simulink model "Hexacopter_ControllerWithNavigation_ver2023b"  (R2023b)
settings: Solver=FixedStepAuto  StartTime=0.0  StopTime=inf  FixedStep=SampleTime  RelTol=1e-3  EnableMultiTasking=on
values from neighbouring files (symbols this model uses):
  SampleTime = 1/250    (= 0.004)    [Init_FLIGHT_Hexacopter.m]    (also in Init_FLIGHT_Hexacopter_fromNCMS.m = 0.01)
undefined symbols (not defined in the file or in its folder): dev, Main, pwm_output0
libraries: px4lib x15, slpidlib x10, px4uORBlib x7, simulink x6, uavalgslib x3, px4Sensorslib x1, simulink_extras x1, sharedutil x1, sharedtransform x1
(part 1 of 3)
settings Model: ExtModeTrigDuration=10  Creator=The MathWorks, Inc.  LastModifiedBy=CNU_UASG
settings SolverCC: PositivePriorityOrder=on  MaxZcPerStep=1
settings OptimizationCC: EnhancedBackFolding=on  PassReuseOutputArgsAs=Individual arguments  ZeroExternalMemoryAtStartup=off  ZeroInternalMemoryAtStartup=off  MaxStackSize=64  OptimizeBlockOrder=speed  DifferentSizesBufferReuse=on  OptimizationCustomize=off  EfficientTunableParamExpr=on
settings DebuggingCC: ParameterTunabilityLossMsg=error
settings HardwareCC: ProdBitPerPointer=32  ProdBitPerSizeT=32  ProdBitPerPtrDiffT=32  ProdLargestAtomicInteger=Long  ProdLargestAtomicFloat=Double  ProdWordSize=32  ProdLongLongMode=on  ProdHWDeviceType=ARM Compatible->ARM Cortex
settings ModelReferenceCC: EnableRefExpFcnMdlSchedulingChecks=on
settings SFSimCC: MATLABDynamicMemAlloc=off  SimTargetLang=C++
settings RTWCC: Description=Embedded Coder  SystemTargetFile=ert.tlc  HardwareBoard=PX4 Cube Orange  TLCOptions="-aInlineSetEventsForThisBaseRateFcn=TLC_FALSE -aSuppressMultiTaskScheduler=TLC_FALSE  -aRateBasedStepFcn=0"  TemplateMakefile=ert_default_tmf  Toolchain=GNU Tools for PX4 Autopilots  TargetLang=C++  DLArmComputeVersion=19.05
settings CodeAppCC: ForceParamTrailComments=on  IgnoreCustomStorageClasses=off  MaxIdLength=63  OperatorAnnotations=on  SimulinkDataObjDesc=on  SFDataObjDesc=on  InsertBlockDesc=on
settings ERTTargetCC: ExtModeTransport=3  ExtModeStaticAlloc=on  ExtModeStaticAllocSize=1024  ExtModeMexFile=ext_xcp  ExtModeIntrfLevel=Level2 - Open

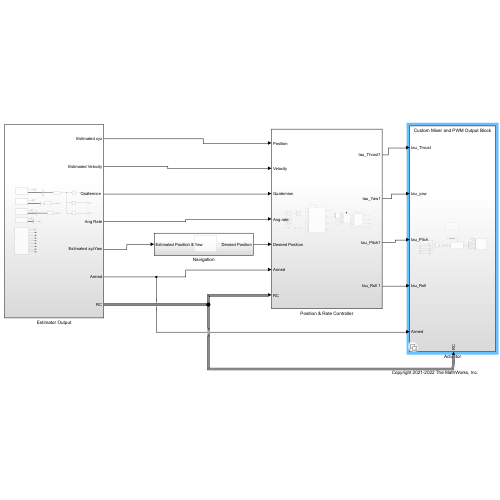
[thumbnail: Simulink's stored preview of the top-level diagram]
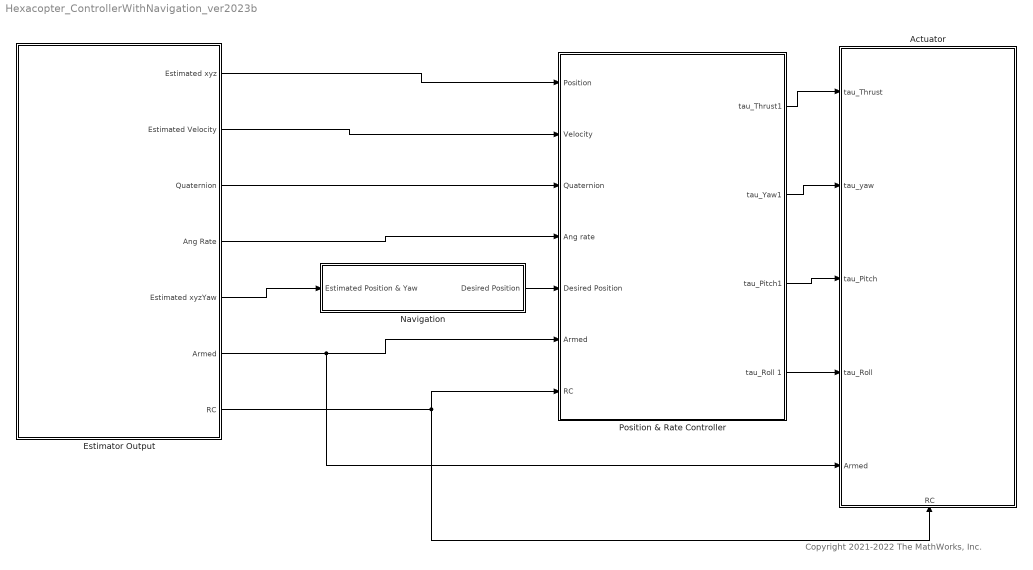
== system Hexacopter_ControllerWithNavigation_ver2023b ==
  note: Copyright 2021-2022 The MathWorks, Inc.
  Actuator : Subsystem  Variant=on
      settings: PortSchema="{\"entries\":[{\"content\":{\"sides\":[{\"content\":{\"connectorIds\":[\"In1\",\"In2\",\"In3\",\"In4\",\"In5\"]},\"type\":\"ConnectorPlacement.EquallySpacedRectSide\",\"uuid\":\"5a9837dd-d0dc-473a-905d-7f1d1e549a1a\"},{\"content\":{\"side\":\"RIGHT\"},\"type\":\"ConnectorPlacement.EquallySpacedRectSide\",\"uuid\":\"ecb902ea-071f-46c7-81c5-182cd0cdfd3c\"},{\"content\":{\"side\":\"TOP\"},\"type\":\"ConnectorPlacement.EquallySpacedRectSide\",\"uuid\":\"3b1ea95c-6dd7-4c60-bfc7-61bcfb955eaa\"},{\"content\":{\"connectorIds\":[\"In6\"],\"side\":\"BOTTOM\"},\"type\":\"ConnectorPlacement.EquallySpacedRectSide\",\"uuid\":\"a3e03740-71d2-4835-8bf3-0b2d7155def1\"}]},\"type\":\"ConnectorPlacement.EquallySpacedConnector\",\"uuid\":\"f571d687-1aa1-4d6b-839e-8b65b8d2b1ab\"}],\"packageUris\":[\"http://schema.mathworks.com/mf0/Connector/R2020b\"],\"version\":\"1.0\"}"
  Estimator Output : Subsystem
  Navigation : Subsystem
  Position & Rate Controller : Subsystem
  wires:
  Estimator Output/5(Estimated xyzYaw) -> Navigation/1(Estimated Position & Yaw)
  Estimator Output/1(Estimated xyz) -> Position & Rate Controller/1(Position)
  Estimator Output/6(Armed) -> Position & Rate Controller/6(Armed), Actuator/5(Armed)
  Estimator Output/2(Estimated Velocity) -> Position & Rate Controller/2(Velocity)
  Estimator Output/7(RC) -> Position & Rate Controller/7(RC), Actuator/6(RC)
  Estimator Output/3("Quaternion ") -> Position & Rate Controller/3(Quaternion)
  Position & Rate Controller/4(tau_Roll 1) -> Actuator/4(tau_Roll)
  Estimator Output/4(Ang Rate) -> Position & Rate Controller/4(Ang rate)
  Navigation/1(Desired Position) -> Position & Rate Controller/5(Desired Position)
  Position & Rate Controller/1(tau_Thrust1) -> Actuator/1(tau_Thrust)
  Position & Rate Controller/2(tau_Yaw1) -> Actuator/2(tau_yaw)
  Position & Rate Controller/3(tau_Pitch1) -> Actuator/3(tau_Pitch)

== system Hexacopter_ControllerWithNavigation_ver2023b/Actuator ==
  tau_Thrust : Inport
  tau_yaw : Inport  Port=2
  tau_Pitch : Inport  Port=3
  tau_Roll : Inport  Port=4
  Armed : Inport  Port=5
  RC : Inport  Port=6
  Custom Mixer and PWM Output Block : Subsystem  VariantControl=useCustomMixer == true
  PX4 Mixer and actuator_controls_0 topic : Subsystem  VariantControl=useCustomMixer == false

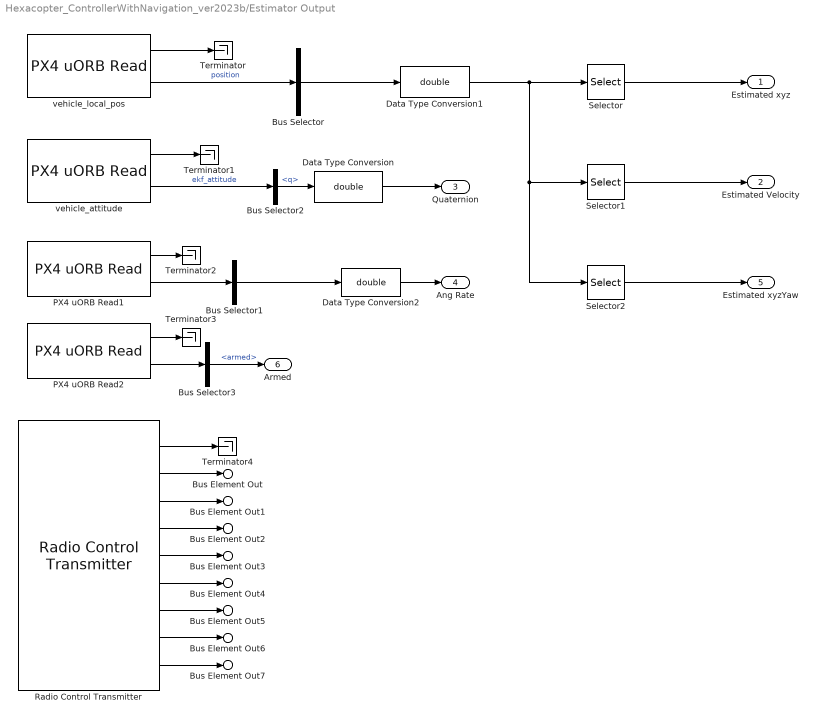
== system Hexacopter_ControllerWithNavigation_ver2023b/Estimator Output ==
  Bus Selector : BusSelector  OutputSignals=x,y,z,vx,vy,vz,heading  OutputAsBus=on
  Bus Selector1 : BusSelector  OutputSignals=rollspeed,pitchspeed,yawspeed  OutputAsBus=on
  Bus Selector2 : BusSelector  OutputSignals=q
  Bus Selector3 : BusSelector  OutputSignals=armed
  Data Type Conversion : DataTypeConversion  OutDataTypeStr=double  SaturateOnIntegerOverflow=off  RndMeth=Floor
  Data Type Conversion1 : DataTypeConversion  OutDataTypeStr=double  SaturateOnIntegerOverflow=off  RndMeth=Floor
  Data Type Conversion2 : DataTypeConversion  OutDataTypeStr=double  SaturateOnIntegerOverflow=off  RndMeth=Floor
  PX4 uORB Read1 : px4uORBlib/PX4 uORB Read  uORBTopic=vehicle_odometry  selectInstance=vehicle_odometry  SampleTime=-1  BlockingMode=off  BlockTimeout=1e-3
  PX4 uORB Read2 : px4uORBlib/PX4 uORB Read  uORBTopic=actuator_armed  selectInstance=actuator_armed  SampleTime=-1  BlockingMode=off  BlockTimeout=1e-3
  Radio Control Transmitter : px4Sensorslib/Radio Control Transmitter  channel1=on  channel2=on  channel3=on  channel4=on  channel5=on  channel6=on  channel7=on  channel8=on  channel_count=off  rssi=off  rc_input_source=off  timestamp_last_signal=off  time_stamp=off  sampleTime=-1  BlockingMode=off  BlockTimeout=5
  Selector : Selector  InputPortWidth=7  IndexOptions=Index vector (dialog)  Indices=[1:3]  OutputSizes=1
  Selector1 : Selector  InputPortWidth=7  IndexOptions=Index vector (dialog)  Indices=[4:6]  OutputSizes=1
  Selector2 : Selector  InputPortWidth=7  IndexOptions=Index vector (dialog)  Indices=[1 2 3 7]  OutputSizes=1
  Terminator{,1..4} (5 alike) : Terminator
  vehicle_attitude : px4uORBlib/PX4 uORB Read  uORBTopic=vehicle_attitude  selectInstance=vehicle_attitude  SampleTime=-1  BlockingMode=off  BlockTimeout=1e-3
  vehicle_local_pos : px4uORBlib/PX4 uORB Read  uORBTopic=vehicle_local_position  selectInstance=vehicle_local_position  SampleTime=-1  BlockingMode=off  BlockTimeout=1e-3
  Estimated xyz : Outport
  Estimated Velocity : Outport  Port=2
  "Quaternion " : Outport  Port=3
  Ang Rate : Outport  Port=4
  Estimated xyzYaw : Outport  Port=5
  Armed : Outport  Port=6
  Bus Element Out : Outport  Port=7  PortName=RC  Element=roll
  Bus Element Out1 : Outport  Port=7  PortName=RC  Element=pitch
  Bus Element Out2 : Outport  Port=7  PortName=RC  Element=throttle
  Bus Element Out3 : Outport  Port=7  PortName=RC  Element=yaw
  Bus Element Out4 : Outport  Port=7  PortName=RC  Element=arm
  Bus Element Out5 : Outport  Port=7  PortName=RC  Element=mode
  Bus Element Out6 : Outport  Port=7  PortName=RC  Element=kill
  Bus Element Out7 : Outport  Port=7  PortName=RC  Element=injectFault
  wires:
  Data Type Conversion/1 -> "Quaternion "/1
  Bus Selector2/1 -> Data Type Conversion/1  "<q>"
  vehicle_local_pos/2 -> Bus Selector/1  "position"
  Data Type Conversion1/1 -> Selector1/1, Selector2/1, Selector/1
  Selector2/1 -> Estimated xyzYaw/1
  vehicle_attitude/1 -> Terminator1/1
  vehicle_attitude/2 -> Bus Selector2/1  "ekf_attitude"
  vehicle_local_pos/1 -> Terminator/1
  Selector/1 -> Estimated xyz/1
  Selector1/1 -> Estimated Velocity/1
  Bus Selector/1 -> Data Type Conversion1/1
  PX4 uORB Read1/1 -> Terminator2/1
  Data Type Conversion2/1 -> Ang Rate/1
  PX4 uORB Read1/2 -> Bus Selector1/1
  PX4 uORB Read2/1 -> Terminator3/1
  Bus Selector3/1 -> Armed/1  "<armed>"
  PX4 uORB Read2/2 -> Bus Selector3/1
  Bus Selector1/1 -> Data Type Conversion2/1
  Radio Control Transmitter/1 -> Terminator4/1
  Radio Control Transmitter/2 -> Bus Element Out/1
  Radio Control Transmitter/3 -> Bus Element Out1/1
  Radio Control Transmitter/4 -> Bus Element Out2/1
  Radio Control Transmitter/5 -> Bus Element Out3/1
  Radio Control Transmitter/6 -> Bus Element Out4/1
  Radio Control Transmitter/7 -> Bus Element Out5/1
  Radio Control Transmitter/8 -> Bus Element Out6/1
  Radio Control Transmitter/9 -> Bus Element Out7/1

== system Hexacopter_ControllerWithNavigation_ver2023b/Navigation ==
  Estimated Position & Yaw : Inport
  Quadcopter Navigation Algorithm : Subsystem  Variant=on
  Desired Position : Outport
  wires:
  Quadcopter Navigation Algorithm/1(Desired Position) -> Desired Position/1
  Estimated Position & Yaw/1 -> Quadcopter Navigation Algorithm/1(Current Position)

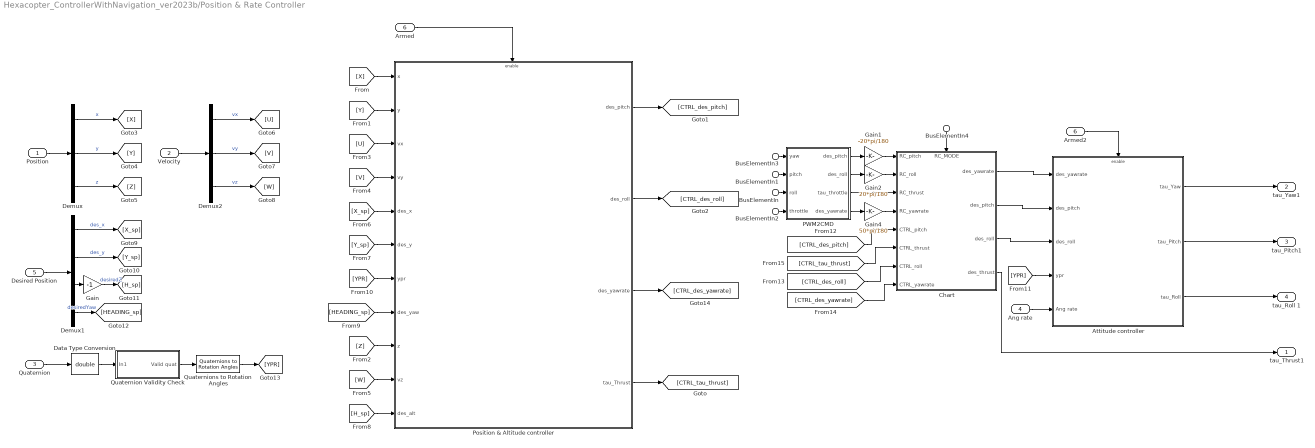
== system Hexacopter_ControllerWithNavigation_ver2023b/Position & Rate Controller ==
  Position : Inport
  Velocity : Inport  Port=2
  Quaternion : Inport  Port=3
  Ang rate : Inport  Port=4
  Desired Position : Inport  Port=5
  Armed : Inport  Port=6
  BusElementIn : Inport  Port=7  PortName=RC  Element=roll
  BusElementIn1 : Inport  Port=7  PortName=RC  Element=pitch
  BusElementIn2 : Inport  Port=7  PortName=RC  Element=throttle
  BusElementIn3 : Inport  Port=7  PortName=RC  Element=yaw
  BusElementIn4 : Inport  Port=7  PortName=RC  Element=mode
  Armed2 : InportShadow  Port=6
  Attitude controller : Subsystem
  Chart : Stateflow chart  TreatAsAtomicUnit=on
      settings: PortSchema="{\"entries\":[{\"content\":{\"sides\":[{\"content\":{\"connectorIds\":[\"In1\",\"In2\",\"In3\",\"In4\",\"In5\",\"In6\",\"In7\",\"In8\"]},\"type\":\"ConnectorPlacement.EquallySpacedRectSide\",\"uuid\":\"1fe492af-6951-4977-8845-2827c5fffa90\"},{\"content\":{\"connectorIds\":[\"Out4\",\"Out1\",\"Out2\",\"Out3\"],\"side\":\"RIGHT\"},\"type\":\"ConnectorPlacement.EquallySpacedRectSide\",\"uuid\":\"b9696a80-46ec-4207-8603-554fdadc7482\"},{\"content\":{\"connectorIds\":[\"In9\"],\"side\":\"TOP\"},\"type\":\"ConnectorPlacement.EquallySpacedRectSide\",\"uuid\":\"36570070-de44-4c7d-99d4-966866a3d58a\"}]},\"type\":\"ConnectorPlacement.EquallySpacedConnector\",\"uuid\":\"856ffff0-a9f0-4cf1-b884-50c3ab6b91f5\"}],\"packageUris\":[\"http://schema.mathworks.com/mf0/Connector/R2020b\"],\"version\":\"1.0\"}"
  Data Type Conversion : DataTypeConversion  OutDataTypeStr=double  SaturateOnIntegerOverflow=off  RndMeth=Floor
  Demux : Demux  Outputs=3
  Demux1 : Demux
  Demux2 : Demux  Outputs=3
  Gain : Gain  Gain=-1
  Gain1 : Gain  Gain=-20*pi/180
  Gain2 : Gain  Gain=20*pi/180
  Gain4 : Gain  Gain=50*pi/180
  PWM2CMD : Subsystem
  Position & Altitude controller : Subsystem
  Quaternion Validity Check : Subsystem
  Quaternions to Rotation Angles : sharedtransform/Quaternions to Rotation Angles  rotationOrder=ZYX  aMode=aMode
  tau_Thrust1 : Outport
  tau_Yaw1 : Outport  Port=2
  tau_Pitch1 : Outport  Port=3
  tau_Roll 1 : Outport  Port=4
  wires:
  Attitude controller/1(tau_Yaw) -> tau_Yaw1/1
  Position & Altitude controller/1(des_pitch) -> [CTRL_des_pitch]
  Data Type Conversion/1 -> Quaternion Validity Check/1(In1)
  Quaternion Validity Check/1(Valid quat) -> Quaternions to Rotation Angles/1
  Position/1 -> Demux/1
  Desired Position/1 -> Demux1/1
  Velocity/1 -> Demux2/1
  Quaternion/1 -> Data Type Conversion/1
  Attitude controller/2(tau_Pitch) -> tau_Pitch1/1
  Attitude controller/3(tau_Roll) -> tau_Roll 1/1
  Demux1/3 -> Gain/1
  Position & Altitude controller/2(des_roll) -> [CTRL_des_roll]
  Ang rate/1 -> Attitude controller/5(Ang rate)
  Demux/1 -> [X]  "x"
  Demux/2 -> [Y]  "y"
  Demux/3 -> [Z]  "z"
  [Y] -> Position & Altitude controller/2(y)
  [X] -> Position & Altitude controller/1(x)
  Demux2/1 -> [U]  "vx"
  Demux2/2 -> [V]  "vy"
  Demux2/3 -> [W]  "vz"
  [U] -> Position & Altitude controller/3(vx)
  [V] -> Position & Altitude controller/4(vy)
  Demux1/1 -> [X_sp]  "des_x"
  Demux1/2 -> [Y_sp]  "des_y"
  Gain/1 -> [H_sp]  "desiredZ"
  [Y_sp] -> Position & Altitude controller/6(des_y)
  [X_sp] -> Position & Altitude controller/5(des_x)
  Demux1/4 -> [HEADING_sp]  "desiredYaw"
  [HEADING_sp] -> Position & Altitude controller/8(des_yaw)
  Quaternions to Rotation Angles/1 -> [YPR]
  [YPR] -> Position & Altitude controller/7(ypr)
  [YPR] -> Attitude controller/4(ypr)
  Position & Altitude controller/3(des_yawrate) -> [CTRL_des_yawrate]
  Chart/4(des_yawrate) -> Attitude controller/1(des_yawrate)
  Chart/1(des_pitch) -> Attitude controller/2(des_pitch)
  Chart/2(des_roll) -> Attitude controller/3(des_roll)
  Chart/3(des_thrust) -> tau_Thrust1/1
  [Z] -> Position & Altitude controller/9(z)
  [W] -> Position & Altitude controller/10(vz)
  [H_sp] -> Position & Altitude controller/11(des_alt)
  Position & Altitude controller/4(tau_Thrust) -> [CTRL_tau_thrust]
  [CTRL_des_pitch] -> Chart/5(CTRL_pitch)
  [CTRL_des_roll] -> Chart/7(CTRL_roll)
  [CTRL_des_yawrate] -> Chart/8(CTRL_yawrate)
  [CTRL_tau_thrust] -> Chart/6(CTRL_thrust)
  BusElementIn3/1 -> PWM2CMD/1(yaw)
  BusElementIn1/1 -> PWM2CMD/2(pitch)
  BusElementIn/1 -> PWM2CMD/3(roll)
  BusElementIn2/1 -> PWM2CMD/4(throttle)
  BusElementIn4/1 -> Chart/9(RC_MODE)
  PWM2CMD/1(des_pitch) -> Gain1/1
  PWM2CMD/4(des_yawrate) -> Gain4/1
  Gain1/1 -> Chart/1(RC_pitch)
  PWM2CMD/3(tau_throttle) -> Chart/3(RC_thrust)
  Gain4/1 -> Chart/4(RC_yawrate)
  PWM2CMD/2(des_roll) -> Gain2/1
  Gain2/1 -> Chart/2(RC_roll)
  Armed/1 -> Position & Altitude controller/Enable
  Armed2/1 -> Attitude controller/Enable

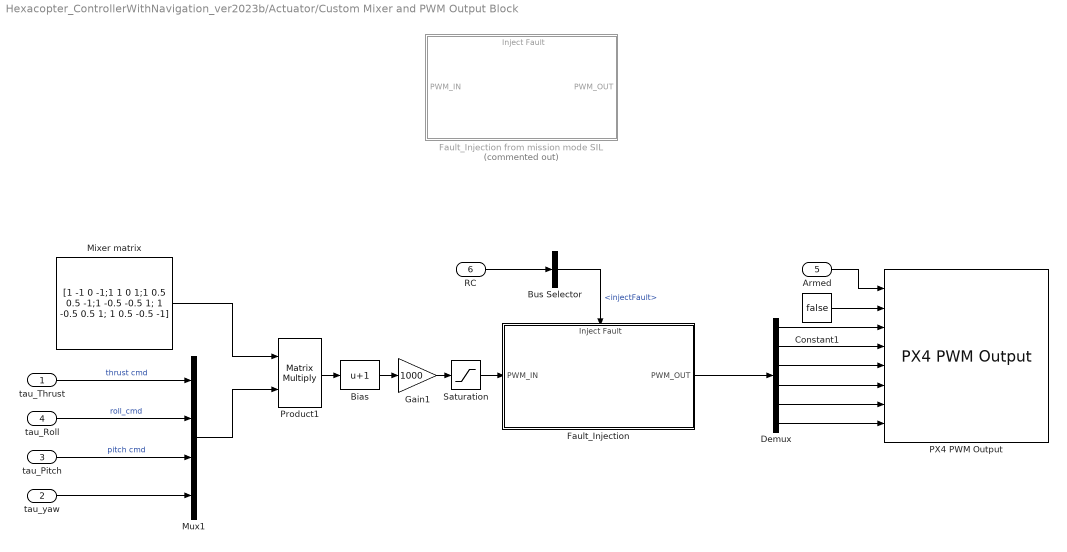
== system Hexacopter_ControllerWithNavigation_ver2023b/Actuator/Custom Mixer and PWM Output Block ==
  tau_Thrust : Inport
  tau_yaw : Inport  Port=2
  tau_Pitch : Inport  Port=3
  tau_Roll : Inport  Port=4
  Armed : Inport  Port=5
  RC : Inport  Port=6
  Bias : Bias  Bias=1  SaturateOnIntegerOverflow=off
  Bus Selector : BusSelector  OutputSignals=injectFault
  Constant1 : Constant  Value=false
  Demux : Demux  Outputs=6
  Fault_Injection : Subsystem  VariantControl=(default)
      settings: PortSchema="{\"entries\":[{\"content\":{\"sides\":[{\"content\":{\"connectorIds\":[\"In1\"]},\"type\":\"ConnectorPlacement.EquallySpacedRectSide\",\"uuid\":\"fab26c65-8d77-46b7-b375-2033d08e8306\"},{\"content\":{\"connectorIds\":[\"Out1\"],\"side\":\"RIGHT\"},\"type\":\"ConnectorPlacement.EquallySpacedRectSide\",\"uuid\":\"bc3f50bd-e170-4b75-8089-4f92da68e83e\"},{\"content\":{\"connectorIds\":[\"In2\"],\"side\":\"TOP\"},\"type\":\"ConnectorPlacement.EquallySpacedRectSide\",\"uuid\":\"873ada90-6f93-48ab-a701-a52d28357753\"}]},\"type\":\"ConnectorPlacement.EquallySpacedConnector\",\"uuid\":\"201be8b3-bff4-4924-8e0c-28e5fee33d1c\"}],\"packageUris\":[\"http://schema.mathworks.com/mf0/Connector/R2020b\"],\"version\":\"1.0\"}"
  Fault_Injection from mission mode SIL : Subsystem  Commented=on
      settings: PortSchema="{\"entries\":[{\"content\":{\"sides\":[{\"content\":{\"connectorIds\":[\"In1\"]},\"type\":\"ConnectorPlacement.EquallySpacedRectSide\",\"uuid\":\"fab26c65-8d77-46b7-b375-2033d08e8306\"},{\"content\":{\"connectorIds\":[\"Out1\"],\"side\":\"RIGHT\"},\"type\":\"ConnectorPlacement.EquallySpacedRectSide\",\"uuid\":\"bc3f50bd-e170-4b75-8089-4f92da68e83e\"},{\"content\":{\"connectorIds\":[\"In2\"],\"side\":\"TOP\"},\"type\":\"ConnectorPlacement.EquallySpacedRectSide\",\"uuid\":\"873ada90-6f93-48ab-a701-a52d28357753\"}]},\"type\":\"ConnectorPlacement.EquallySpacedConnector\",\"uuid\":\"201be8b3-bff4-4924-8e0c-28e5fee33d1c\"}],\"packageUris\":[\"http://schema.mathworks.com/mf0/Connector/R2020b\"],\"version\":\"1.0\"}"
  Gain1 : Gain  Gain=1000  OutDataTypeStr=uint16
  Mixer matrix : Constant  Value=[1 -1 0 -1;1 1 0 1;1 0.5 0.5 -1;1 -0.5 -0.5 1; 1 -0.5 0.5 1; 1 0.5 -0.5 -1]  OutDataTypeStr=Inherit: Inherit via back propagation  SampleTime=-1
  Mux1 : Mux
  PX4 PWM Output : px4lib/PX4 PWM Output  pwmDevice=Main (/dev/pwm_output0)  pwmChannel1_=on  pwmChannel2_=on  pwmChannel3_=on  pwmChannel4_=on  pwmChannel5_=on  pwmChannel6_=on  pwmChannel7_=off  pwmChannel8_=off  forceTerminateFailsafe=off  outputErrorStatus=off
  Product1 : Product  Multiplication=Matrix(*)  RndMeth=Zero
  Saturation : Saturate  UpperLimit=2000  LowerLimit=1000
  wires:
  Demux/1 -> PX4 PWM Output/3
  Demux/2 -> PX4 PWM Output/4
  Gain1/1 -> Saturation/1
  Mux1/1 -> Product1/2
  Mixer matrix/1 -> Product1/1
  tau_Thrust/1 -> Mux1/1  "thrust cmd"
  Constant1/1 -> PX4 PWM Output/2
  Demux/3 -> PX4 PWM Output/5
  Armed/1 -> PX4 PWM Output/1
  Product1/1 -> Bias/1
  Demux/4 -> PX4 PWM Output/6
  Bias/1 -> Gain1/1
  tau_Roll/1 -> Mux1/2  "roll_cmd"
  tau_Pitch/1 -> Mux1/3  "pitch cmd"
  tau_yaw/1 -> Mux1/4
  Demux/5 -> PX4 PWM Output/7
  Demux/6 -> PX4 PWM Output/8
  RC/1 -> Bus Selector/1
  Saturation/1 -> Fault_Injection/1(PWM_IN)
  Fault_Injection/1(PWM_OUT) -> Demux/1
  Bus Selector/1 -> Fault_Injection/2(Inject Fault)  "<injectFault>"

== system Hexacopter_ControllerWithNavigation_ver2023b/Actuator/PX4 Mixer and actuator_controls_0 topic ==
  tau_Thrust : Inport
  tau_yaw : Inport  Port=2
  tau_Pitch : Inport  Port=3
  tau_Roll : Inport  Port=4
  Armed : Inport  Port=5
  RC : Inport  Port=6
  Bus Assignment : BusAssignment  AssignedSignals=control
  Constant : Constant  Value=zeros(4,1)
  Data Type Conversion : DataTypeConversion  SaturateOnIntegerOverflow=off  RndMeth=Floor
  Mux : Mux  Inputs=5
  PX4 uORB Message : px4uORBlib/PX4 uORB Message  uORBTopic=actuator_controls  SampleTime=inf  selectInstance=vehicle_gps_position
  PX4 uORB Write : px4uORBlib/PX4 uORB Write  uORBTopic=actuator_controls  selectInstance=actuator_controls_0  MessageQueueLen=1
  Terminator : Terminator
  wires:
  Bus Assignment/1 -> PX4 uORB Write/1
  tau_yaw/1 -> Mux/3
  Data Type Conversion/1 -> Bus Assignment/2
  tau_Roll/1 -> Mux/1  "roll_cmd"
  PX4 uORB Message/1 -> Bus Assignment/1
  Mux/1 -> Data Type Conversion/1
  Constant/1 -> Mux/5
  tau_Pitch/1 -> Mux/2  "pitch cmd"
  tau_Thrust/1 -> Mux/4  "thrust cmd"
  Armed/1 -> Terminator/1

== system Hexacopter_ControllerWithNavigation_ver2023b/Navigation/Quadcopter Navigation Algorithm ==
  Current Position : Inport
  Manual Waypoints : Subsystem  VariantControl=guidanceType == 3
  Manual Waypoints from Simulink Dashboard : Subsystem  VariantControl=guidanceType == 2
  Path Correction from Onboard Computer : Subsystem  VariantControl=guidanceType == 1
  Read waypoint from QGroundControl Mission : Subsystem  VariantControl=guidanceType == 0
  Desired Position : Outport

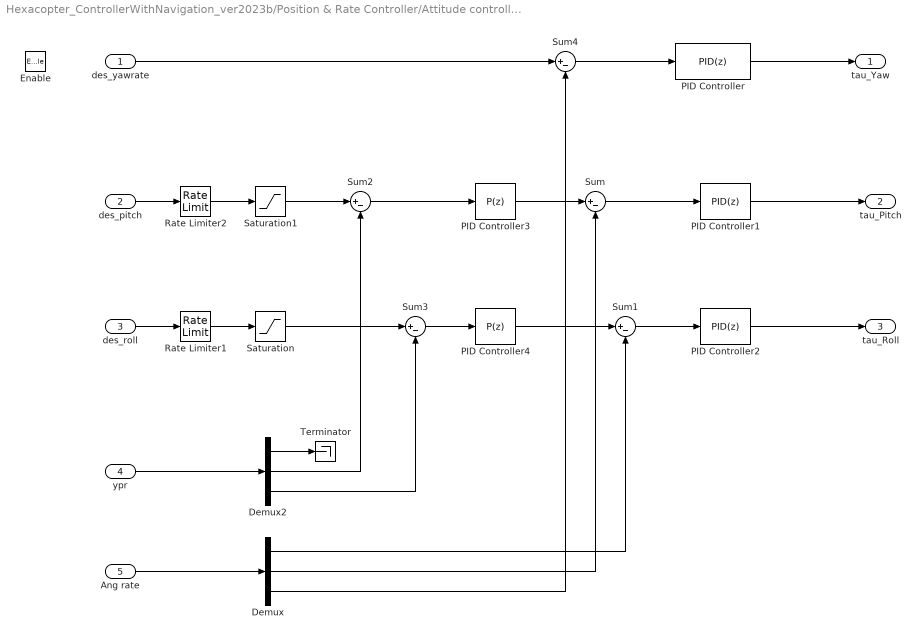
== system Hexacopter_ControllerWithNavigation_ver2023b/Position & Rate Controller/Attitude controller ==
  des_yawrate : Inport
  des_pitch : Inport  Port=2
  des_roll : Inport  Port=3
  ypr : Inport  Port=4
  Ang rate : Inport  Port=5
  Enable : EnablePort
  Demux : Demux  Outputs=3
  Demux2 : Demux  Outputs=3
  PID Controller : slpidlib/PID Controller  Controller=PID  Form=Parallel  TimeDomain=Discrete-time  UseExternalTs=off  SampleTime=-1  IntegratorMethod=Forward Euler  FilterMethod=Forward Euler  ControllerParametersSource=internal  P=0.2/10  I=0.1/10  UseKiTs=on  D=0  N=100  UseFilter=on  TunerSelectOption=Transfer Function Based (PID Tuner App)  InitialConditionSource=internal  InitialConditionForIntegrator=0  InitialConditionForFilter=0  DifferentiatorICPrevScaledInput=0  ExternalReset=none  TrackingMode=off  Kt=1  LimitOutput=on  SatLimitsSource=internal  UpperSaturationLimit=0.1  LowerSaturationLimit=-0.1  LinearizeAsGain=on  AntiWindupMode=clamping  Kb=1  LimitIntegrator=off  UpperIntegratorSaturationLimit=inf  LowerIntegratorSaturationLimit=-inf  POutMin=[]  POutMax=[]  IOutMin=[]  IOutMax=[]  DOutMin=[]  DOutMax=[]  NOutMin=[]  NOutMax=[]  SumOutMin=[]  SumOutMax=[]  SaturationOutMin=[]  SaturationOutMax=[]  PParamMin=[]  PParamMax=[]  IParamMin=[]  IParamMax=[]  DParamMin=[]  DParamMax=[]  NParamMin=[]  NParamMax=[]  KbParamMin=[]  KbParamMax=[]  KtParamMin=[]  KtParamMax=[]  KbOutMin=[]  KbOutMax=[]  KtOutMin=[]  KtOutMax=[]  IntegratorOutMin=[]  IntegratorOutMax=[]  FilterOutMin=[]  FilterOutMax=[]  SumI1OutMin=[]  SumI1OutMax=[]  SumI2OutMin=[]  SumI2OutMax=[]  SumI3OutMin=[]  SumI3OutMax=[]  SumI4OutMin=[]  SumI4OutMax=[]  SumDOutMin=[]  SumDOutMax=[]  DifferentiatorOutMin=[]  DifferentiatorOutMax=[]  FilterDiffOutCoefMin=[]  FilterDiffOutCoefMax=[]  ReciprocalOutMin=[]  ReciprocalOutMax=[]  SumDenOutMin=[]  SumDenOutMax=[]  SumNumOutMin=[]  SumNumOutMax=[]  DivideOutMin=[]  DivideOutMax=[]  UdiffTsProdOutMin=[]  UdiffTsProdOutMax=[]  NTsProdOutMin=[]  NTsProdOutMax=[]  UintegralTsProdOutMin=[]  UintegralTsProdOutMax=[]  UngainTsProdOutMin=[]  UngainTsProdOutMax=[]  ClampingZeroOutDataTypeStr=Inherit: Inherit via back propagation  ClampingZeroOutMin=[]  ClampingZeroOutMax=[]  FilterDenConstantOutDataTypeStr=Inherit: Inherit via back propagation  FilterDenConstantOutMin=[]  FilterDenConstantOutMax=[]  PCopyOutDataTypeStr=Inherit: Inherit via back propagation  PCopyOutMin=[]  PCopyOutMax=[]  NCopyOutDataTypeStr=Inherit: Inherit via back propagation  NCopyOutMin=[]  NCopyOutMax=[]  IntegratorContinuousStateAttributes=''  IntegratorStateMustResolveToSignalObject=off  IntegratorRTWStateStorageClass=Auto  FilterContinuousStateAttributes=''  FilterStateMustResolveToSignalObject=off  FilterRTWStateStorageClass=Auto  ParallelPVariant=InternalParameters  IdealPVariant=Disabled  IVariant=InternalParameters  DVariant=InternalParameters  IntegratorVariant=Discrete  SatVariant=Enabled  AWVariant=DiscClampingParallel  PCopyVariant=Disabled  TRVariant=Disabled  FdbkBlocksVariant=Forward  IdealPFdbkVariant=Disabled  SatFdbkVariant=Disabled  DerivativeFilterVariant=ForwardEulerFilter  NVariant=InternalParameters  NCopyVariant=Disabled  FilterICVariant=InternalICsFilter  IntegratorICVariant=InternalICs  ExternalResetVariant=Disabled  TRSumVariant=Passthrough  SumFdbkVariant=Disabled  SumVariant=Sum_PID  TsampFilterVariant=InternalTs  TsampNgainVariant=Passthrough  TsampIntegralVariant=Disabled_SignalSpec  ExternalSaturationOutDataTypeStr=Inherit: Same as second input
  PID Controller1 : slpidlib/PID Controller  Controller=PID  Form=Parallel  TimeDomain=Discrete-time  UseExternalTs=off  SampleTime=-1  IntegratorMethod=Forward Euler  FilterMethod=Forward Euler  ControllerParametersSource=internal  P=0.15/5  I=0.2/5  UseKiTs=on  D=0.003/5  N=50  UseFilter=on  TunerSelectOption=Transfer Function Based (PID Tuner App)  InitialConditionSource=internal  InitialConditionForIntegrator=0  InitialConditionForFilter=0  DifferentiatorICPrevScaledInput=0  ExternalReset=none  TrackingMode=off  Kt=1  LimitOutput=on  SatLimitsSource=internal  UpperSaturationLimit=0.2  LowerSaturationLimit=-0.2  LinearizeAsGain=on  AntiWindupMode=clamping  Kb=1  LimitIntegrator=off  UpperIntegratorSaturationLimit=inf  LowerIntegratorSaturationLimit=-inf  POutMin=[]  POutMax=[]  IOutMin=[]  IOutMax=[]  DOutMin=[]  DOutMax=[]  NOutMin=[]  NOutMax=[]  SumOutMin=[]  SumOutMax=[]  SaturationOutMin=[]  SaturationOutMax=[]  PParamMin=[]  PParamMax=[]  IParamMin=[]  IParamMax=[]  DParamMin=[]  DParamMax=[]  NParamMin=[]  NParamMax=[]  KbParamMin=[]  KbParamMax=[]  KtParamMin=[]  KtParamMax=[]  KbOutMin=[]  KbOutMax=[]  KtOutMin=[]  KtOutMax=[]  IntegratorOutMin=[]  IntegratorOutMax=[]  FilterOutMin=[]  FilterOutMax=[]  SumI1OutMin=[]  SumI1OutMax=[]  SumI2OutMin=[]  SumI2OutMax=[]  SumI3OutMin=[]  SumI3OutMax=[]  SumI4OutMin=[]  SumI4OutMax=[]  SumDOutMin=[]  SumDOutMax=[]  DifferentiatorOutMin=[]  DifferentiatorOutMax=[]  FilterDiffOutCoefMin=[]  FilterDiffOutCoefMax=[]  ReciprocalOutMin=[]  ReciprocalOutMax=[]  SumDenOutMin=[]  SumDenOutMax=[]  SumNumOutMin=[]  SumNumOutMax=[]  DivideOutMin=[]  DivideOutMax=[]  UdiffTsProdOutMin=[]  UdiffTsProdOutMax=[]  NTsProdOutMin=[]  NTsProdOutMax=[]  UintegralTsProdOutMin=[]  UintegralTsProdOutMax=[]  UngainTsProdOutMin=[]  UngainTsProdOutMax=[]  ClampingZeroOutDataTypeStr=Inherit: Inherit via back propagation  ClampingZeroOutMin=[]  ClampingZeroOutMax=[]  FilterDenConstantOutDataTypeStr=Inherit: Inherit via back propagation  FilterDenConstantOutMin=[]  FilterDenConstantOutMax=[]  PCopyOutDataTypeStr=Inherit: Inherit via back propagation  PCopyOutMin=[]  PCopyOutMax=[]  NCopyOutDataTypeStr=Inherit: Inherit via back propagation  NCopyOutMin=[]  NCopyOutMax=[]  IntegratorContinuousStateAttributes=''  IntegratorStateMustResolveToSignalObject=off  IntegratorRTWStateStorageClass=Auto  FilterContinuousStateAttributes=''  FilterStateMustResolveToSignalObject=off  FilterRTWStateStorageClass=Auto  ParallelPVariant=InternalParameters  IdealPVariant=Disabled  IVariant=InternalParameters  DVariant=InternalParameters  IntegratorVariant=Discrete  SatVariant=Enabled  AWVariant=DiscClampingParallel  PCopyVariant=Disabled  TRVariant=Disabled  FdbkBlocksVariant=Forward  IdealPFdbkVariant=Disabled  SatFdbkVariant=Disabled  DerivativeFilterVariant=ForwardEulerFilter  NVariant=InternalParameters  NCopyVariant=Disabled  FilterICVariant=InternalICsFilter  IntegratorICVariant=InternalICs  ExternalResetVariant=Disabled  TRSumVariant=Passthrough  SumFdbkVariant=Disabled  SumVariant=Sum_PID  TsampFilterVariant=InternalTs  TsampNgainVariant=Passthrough  TsampIntegralVariant=Disabled_SignalSpec  ExternalSaturationOutDataTypeStr=Inherit: Same as second input
  PID Controller2 : slpidlib/PID Controller  Controller=PID  Form=Parallel  TimeDomain=Discrete-time  UseExternalTs=off  SampleTime=-1  IntegratorMethod=Forward Euler  FilterMethod=Forward Euler  ControllerParametersSource=internal  P=0.15/5  I=0.2/5  UseKiTs=off  D=0.003/5  N=50  UseFilter=on  TunerSelectOption=Transfer Function Based (PID Tuner App)  InitialConditionSource=internal  InitialConditionForIntegrator=0  InitialConditionForFilter=0  DifferentiatorICPrevScaledInput=0  ExternalReset=none  TrackingMode=off  Kt=1  LimitOutput=on  SatLimitsSource=internal  UpperSaturationLimit=0.2  LowerSaturationLimit=-0.2  LinearizeAsGain=on  AntiWindupMode=clamping  Kb=1  LimitIntegrator=off  UpperIntegratorSaturationLimit=inf  LowerIntegratorSaturationLimit=-inf  POutMin=[]  POutMax=[]  IOutMin=[]  IOutMax=[]  DOutMin=[]  DOutMax=[]  NOutMin=[]  NOutMax=[]  SumOutMin=[]  SumOutMax=[]  SaturationOutMin=[]  SaturationOutMax=[]  PParamMin=[]  PParamMax=[]  IParamMin=[]  IParamMax=[]  DParamMin=[]  DParamMax=[]  NParamMin=[]  NParamMax=[]  KbParamMin=[]  KbParamMax=[]  KtParamMin=[]  KtParamMax=[]  KbOutMin=[]  KbOutMax=[]  KtOutMin=[]  KtOutMax=[]  IntegratorOutMin=[]  IntegratorOutMax=[]  FilterOutMin=[]  FilterOutMax=[]  SumI1OutMin=[]  SumI1OutMax=[]  SumI2OutMin=[]  SumI2OutMax=[]  SumI3OutMin=[]  SumI3OutMax=[]  SumI4OutMin=[]  SumI4OutMax=[]  SumDOutMin=[]  SumDOutMax=[]  DifferentiatorOutMin=[]  DifferentiatorOutMax=[]  FilterDiffOutCoefMin=[]  FilterDiffOutCoefMax=[]  ReciprocalOutMin=[]  ReciprocalOutMax=[]  SumDenOutMin=[]  SumDenOutMax=[]  SumNumOutMin=[]  SumNumOutMax=[]  DivideOutMin=[]  DivideOutMax=[]  UdiffTsProdOutMin=[]  UdiffTsProdOutMax=[]  NTsProdOutMin=[]  NTsProdOutMax=[]  UintegralTsProdOutMin=[]  UintegralTsProdOutMax=[]  UngainTsProdOutMin=[]  UngainTsProdOutMax=[]  ClampingZeroOutDataTypeStr=Inherit: Inherit via back propagation  ClampingZeroOutMin=[]  ClampingZeroOutMax=[]  FilterDenConstantOutDataTypeStr=Inherit: Inherit via back propagation  FilterDenConstantOutMin=[]  FilterDenConstantOutMax=[]  PCopyOutDataTypeStr=Inherit: Inherit via back propagation  PCopyOutMin=[]  PCopyOutMax=[]  NCopyOutDataTypeStr=Inherit: Inherit via back propagation  NCopyOutMin=[]  NCopyOutMax=[]  IntegratorContinuousStateAttributes=''  IntegratorStateMustResolveToSignalObject=off  IntegratorRTWStateStorageClass=Auto  FilterContinuousStateAttributes=''  FilterStateMustResolveToSignalObject=off  FilterRTWStateStorageClass=Auto  ParallelPVariant=InternalParameters  IdealPVariant=Disabled  IVariant=InternalParameters  DVariant=InternalParameters  IntegratorVariant=Discrete  SatVariant=Enabled  AWVariant=DiscClampingParallel  PCopyVariant=Disabled  TRVariant=Disabled  FdbkBlocksVariant=Forward  IdealPFdbkVariant=Disabled  SatFdbkVariant=Disabled  DerivativeFilterVariant=ForwardEulerFilter  NVariant=InternalParameters  NCopyVariant=Disabled  FilterICVariant=InternalICsFilter  IntegratorICVariant=InternalICs  ExternalResetVariant=Disabled  TRSumVariant=Passthrough  SumFdbkVariant=Disabled  SumVariant=Sum_PID  TsampFilterVariant=InternalTs  TsampNgainVariant=Passthrough  TsampIntegralVariant=Disabled_SignalSpec  ExternalSaturationOutDataTypeStr=Inherit: Same as second input
  PID Controller3 : slpidlib/PID Controller  Controller=P  Form=Parallel  TimeDomain=Discrete-time  UseExternalTs=off  SampleTime=-1  IntegratorMethod=Forward Euler  FilterMethod=Forward Euler  ControllerParametersSource=internal  P=6.5/5  I=1  UseKiTs=off  D=0  N=100  UseFilter=on  TunerSelectOption=Transfer Function Based (PID Tuner App)  InitialConditionSource=internal  InitialConditionForIntegrator=0  InitialConditionForFilter=0  DifferentiatorICPrevScaledInput=0  ExternalReset=none  TrackingMode=off  Kt=1  LimitOutput=off  SatLimitsSource=internal  UpperSaturationLimit=inf  LowerSaturationLimit=-inf  LinearizeAsGain=on  AntiWindupMode=none  Kb=1  LimitIntegrator=off  UpperIntegratorSaturationLimit=inf  LowerIntegratorSaturationLimit=-inf  POutMin=[]  POutMax=[]  IOutMin=[]  IOutMax=[]  DOutMin=[]  DOutMax=[]  NOutMin=[]  NOutMax=[]  SumOutMin=[]  SumOutMax=[]  SaturationOutMin=[]  SaturationOutMax=[]  PParamMin=[]  PParamMax=[]  IParamMin=[]  IParamMax=[]  DParamMin=[]  DParamMax=[]  NParamMin=[]  NParamMax=[]  KbParamMin=[]  KbParamMax=[]  KtParamMin=[]  KtParamMax=[]  KbOutMin=[]  KbOutMax=[]  KtOutMin=[]  KtOutMax=[]  IntegratorOutMin=[]  IntegratorOutMax=[]  FilterOutMin=[]  FilterOutMax=[]  SumI1OutMin=[]  SumI1OutMax=[]  SumI2OutMin=[]  SumI2OutMax=[]  SumI3OutMin=[]  SumI3OutMax=[]  SumI4OutMin=[]  SumI4OutMax=[]  SumDOutMin=[]  SumDOutMax=[]  DifferentiatorOutMin=[]  DifferentiatorOutMax=[]  FilterDiffOutCoefMin=[]  FilterDiffOutCoefMax=[]  ReciprocalOutMin=[]  ReciprocalOutMax=[]  SumDenOutMin=[]  SumDenOutMax=[]  SumNumOutMin=[]  SumNumOutMax=[]  DivideOutMin=[]  DivideOutMax=[]  UdiffTsProdOutMin=[]  UdiffTsProdOutMax=[]  NTsProdOutMin=[]  NTsProdOutMax=[]  UintegralTsProdOutMin=[]  UintegralTsProdOutMax=[]  UngainTsProdOutMin=[]  UngainTsProdOutMax=[]  ClampingZeroOutDataTypeStr=Inherit: Inherit via back propagation  ClampingZeroOutMin=[]  ClampingZeroOutMax=[]  FilterDenConstantOutDataTypeStr=Inherit: Inherit via back propagation  FilterDenConstantOutMin=[]  FilterDenConstantOutMax=[]  PCopyOutDataTypeStr=Inherit: Inherit via back propagation  PCopyOutMin=[]  PCopyOutMax=[]  NCopyOutDataTypeStr=Inherit: Inherit via back propagation  NCopyOutMin=[]  NCopyOutMax=[]  IntegratorContinuousStateAttributes=''  IntegratorStateMustResolveToSignalObject=off  IntegratorRTWStateStorageClass=Auto  FilterContinuousStateAttributes=''  FilterStateMustResolveToSignalObject=off  FilterRTWStateStorageClass=Auto  ParallelPVariant=InternalParameters  IdealPVariant=Disabled  IVariant=Disabled  DVariant=Disabled  IntegratorVariant=Disabled  SatVariant=Disabled  AWVariant=Disabled  PCopyVariant=Disabled  TRVariant=Disabled  FdbkBlocksVariant=Forward  IdealPFdbkVariant=Disabled  SatFdbkVariant=Disabled  DerivativeFilterVariant=Disabled  NVariant=Disabled  NCopyVariant=Disabled_SignalSpec  FilterICVariant=Disabled  IntegratorICVariant=Disabled  ExternalResetVariant=Disabled  TRSumVariant=Passthrough  SumFdbkVariant=Disabled  SumVariant=Passthrough_P  TsampFilterVariant=InternalTs  TsampNgainVariant=Passthrough  TsampIntegralVariant=Disabled_SignalSpec  ExternalSaturationOutDataTypeStr=Inherit: Same as second input
  PID Controller4 : slpidlib/PID Controller  Controller=P  Form=Parallel  TimeDomain=Discrete-time  UseExternalTs=off  SampleTime=-1  IntegratorMethod=Forward Euler  FilterMethod=Forward Euler  ControllerParametersSource=internal  P=4/5  I=1  UseKiTs=off  D=0  N=100  UseFilter=on  TunerSelectOption=Transfer Function Based (PID Tuner App)  InitialConditionSource=internal  InitialConditionForIntegrator=0  InitialConditionForFilter=0  DifferentiatorICPrevScaledInput=0  ExternalReset=none  TrackingMode=off  Kt=1  LimitOutput=off  SatLimitsSource=internal  UpperSaturationLimit=inf  LowerSaturationLimit=-inf  LinearizeAsGain=on  AntiWindupMode=none  Kb=1  LimitIntegrator=off  UpperIntegratorSaturationLimit=inf  LowerIntegratorSaturationLimit=-inf  POutMin=[]  POutMax=[]  IOutMin=[]  IOutMax=[]  DOutMin=[]  DOutMax=[]  NOutMin=[]  NOutMax=[]  SumOutMin=[]  SumOutMax=[]  SaturationOutMin=[]  SaturationOutMax=[]  PParamMin=[]  PParamMax=[]  IParamMin=[]  IParamMax=[]  DParamMin=[]  DParamMax=[]  NParamMin=[]  NParamMax=[]  KbParamMin=[]  KbParamMax=[]  KtParamMin=[]  KtParamMax=[]  KbOutMin=[]  KbOutMax=[]  KtOutMin=[]  KtOutMax=[]  IntegratorOutMin=[]  IntegratorOutMax=[]  FilterOutMin=[]  FilterOutMax=[]  SumI1OutMin=[]  SumI1OutMax=[]  SumI2OutMin=[]  SumI2OutMax=[]  SumI3OutMin=[]  SumI3OutMax=[]  SumI4OutMin=[]  SumI4OutMax=[]  SumDOutMin=[]  SumDOutMax=[]  DifferentiatorOutMin=[]  DifferentiatorOutMax=[]  FilterDiffOutCoefMin=[]  FilterDiffOutCoefMax=[]  ReciprocalOutMin=[]  ReciprocalOutMax=[]  SumDenOutMin=[]  SumDenOutMax=[]  SumNumOutMin=[]  SumNumOutMax=[]  DivideOutMin=[]  DivideOutMax=[]  UdiffTsProdOutMin=[]  UdiffTsProdOutMax=[]  NTsProdOutMin=[]  NTsProdOutMax=[]  UintegralTsProdOutMin=[]  UintegralTsProdOutMax=[]  UngainTsProdOutMin=[]  UngainTsProdOutMax=[]  ClampingZeroOutDataTypeStr=Inherit: Inherit via back propagation  ClampingZeroOutMin=[]  ClampingZeroOutMax=[]  FilterDenConstantOutDataTypeStr=Inherit: Inherit via back propagation  FilterDenConstantOutMin=[]  FilterDenConstantOutMax=[]  PCopyOutDataTypeStr=Inherit: Inherit via back propagation  PCopyOutMin=[]  PCopyOutMax=[]  NCopyOutDataTypeStr=Inherit: Inherit via back propagation  NCopyOutMin=[]  NCopyOutMax=[]  IntegratorContinuousStateAttributes=''  IntegratorStateMustResolveToSignalObject=off  IntegratorRTWStateStorageClass=Auto  FilterContinuousStateAttributes=''  FilterStateMustResolveToSignalObject=off  FilterRTWStateStorageClass=Auto  ParallelPVariant=InternalParameters  IdealPVariant=Disabled  IVariant=Disabled  DVariant=Disabled  IntegratorVariant=Disabled  SatVariant=Disabled  AWVariant=Disabled  PCopyVariant=Disabled  TRVariant=Disabled  FdbkBlocksVariant=Forward  IdealPFdbkVariant=Disabled  SatFdbkVariant=Disabled  DerivativeFilterVariant=Disabled  NVariant=Disabled  NCopyVariant=Disabled_SignalSpec  FilterICVariant=Disabled  IntegratorICVariant=Disabled  ExternalResetVariant=Disabled  TRSumVariant=Passthrough  SumFdbkVariant=Disabled  SumVariant=Passthrough_P  TsampFilterVariant=InternalTs  TsampNgainVariant=Passthrough  TsampIntegralVariant=Disabled_SignalSpec  ExternalSaturationOutDataTypeStr=Inherit: Same as second input
  Rate Limiter1 : RateLimiter  RisingSlewLimit=180*pi/180  FallingSlewLimit=-180*pi/180  SampleTimeMode=inherited
  Rate Limiter2 : RateLimiter  RisingSlewLimit=180*pi/180  FallingSlewLimit=-180*pi/180  SampleTimeMode=inherited
  Saturation : Saturate  UpperLimit=20*pi/180  LowerLimit=-20*pi/180
  Saturation1 : Saturate  UpperLimit=20*pi/180  LowerLimit=-20*pi/180
  Sum{,1..4} (5 alike) : Sum  Inputs=|+-
  Terminator : Terminator
  tau_Yaw : Outport
  tau_Pitch : Outport  Port=2
  tau_Roll : Outport  Port=3
  wires:
  PID Controller/1 -> tau_Yaw/1
  Sum/1 -> PID Controller1/1
  Ang rate/1 -> Demux/1
  Demux/2 -> Sum/2
  PID Controller1/1 -> tau_Pitch/1
  Sum1/1 -> PID Controller2/1
  Demux/1 -> Sum1/2
  PID Controller2/1 -> tau_Roll/1
  Sum2/1 -> PID Controller3/1
  Sum3/1 -> PID Controller4/1
  ypr/1 -> Demux2/1
  Demux2/2 -> Sum2/2
  Demux2/3 -> Sum3/2
  Sum4/1 -> PID Controller/1
  Demux/3 -> Sum4/2
  des_roll/1 -> Rate Limiter1/1
  Rate Limiter1/1 -> Saturation/1
  Rate Limiter2/1 -> Saturation1/1
  Saturation/1 -> Sum3/1
  PID Controller3/1 -> Sum/1
  Saturation1/1 -> Sum2/1
  des_pitch/1 -> Rate Limiter2/1
  PID Controller4/1 -> Sum1/1
  Demux2/1 -> Terminator/1
  des_yawrate/1 -> Sum4/1

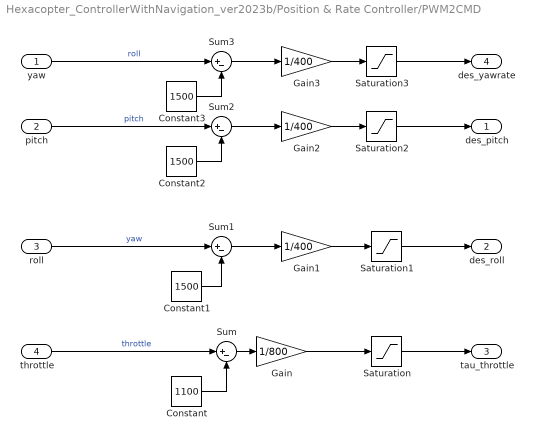
== system Hexacopter_ControllerWithNavigation_ver2023b/Position & Rate Controller/PWM2CMD ==
  yaw : Inport
  pitch : Inport  Port=2
  roll : Inport  Port=3
  throttle : Inport  Port=4
  Constant : Constant  Value=1100
  Constant1 : Constant  Value=1500
  Constant2 : Constant  Value=1500
  Constant3 : Constant  Value=1500
  Gain : Gain  Gain=1/800
  Gain1 : Gain  Gain=1/400
  Gain2 : Gain  Gain=1/400
  Gain3 : Gain  Gain=1/400
  Saturation : Saturate  UpperLimit=0.90  LowerLimit=0
  Saturation1 : Saturate  UpperLimit=1  LowerLimit=-1
  Saturation2 : Saturate  UpperLimit=1  LowerLimit=-1
  Saturation3 : Saturate  UpperLimit=1  LowerLimit=-1
  Sum{,1..3} (4 alike) : Sum  Inputs=|+-
  des_pitch : Outport
  des_roll : Outport  Port=2
  tau_throttle : Outport  Port=3
  des_yawrate : Outport  Port=4
  wires:
  Gain/1 -> Saturation/1
  Constant1/1 -> Sum1/2
  throttle/1 -> Sum/1  "throttle"
  yaw/1 -> Sum3/1  "roll"
  Constant3/1 -> Sum3/2
  Gain2/1 -> Saturation2/1
  pitch/1 -> Sum2/1  "pitch"
  Constant2/1 -> Sum2/2
  roll/1 -> Sum1/1  "yaw"
  Sum1/1 -> Gain1/1
  Sum2/1 -> Gain2/1
  Gain3/1 -> Saturation3/1
  Constant/1 -> Sum/2
  Sum/1 -> Gain/1
  Sum3/1 -> Gain3/1
  Gain1/1 -> Saturation1/1
  Saturation3/1 -> des_yawrate/1
  Saturation2/1 -> des_pitch/1
  Saturation1/1 -> des_roll/1
  Saturation/1 -> tau_throttle/1
